simulink model "QPSK1"  (Simulink 8.0)
settings: Solver=ode45  StartTime=0.0  StopTime=12  RelTol=1e-3
libraries: commsequence2 x1, commseqgen2 x1, commutil2 x1
settings Model: Creator=Dimav  LastModifiedBy=Dimav

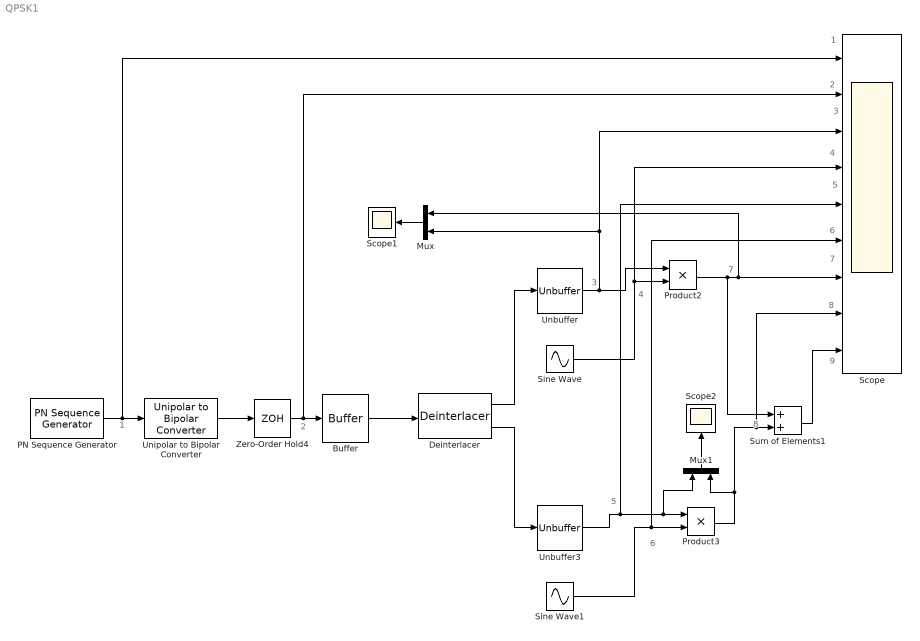
== system QPSK1 ==
  note: 8
  note: 5
  note: 5
  note: 6
  note: 6
  note: 7
  note: 7
  note: 3
  note: 4
  note: 2
  note: 1
  note: 3
  note: 8
  note: 9
  note: 1
  note: 2
  note: 4
  Buffer : Buffer  N=2  TreatMby1Signals=One channel
  Deinterlacer : commsequence2/Deinterlacer
  Mux : Mux  Inputs=2
  Mux1 : Mux  Inputs=2
  PN Sequence Generator : commseqgen2/PN Sequence Generator  poly=[1 0 0 0 0 1 1]  ini_sta=[0 0 0 0 0 1]  outBitMaskSource=Dialog parameter  shift=0  outVarSiz=off  maxOutSizeMode=Dialog parameter  maxOutSize=[10 1]  Ts=1/1200  frameBased=off  sampPerFrame=1  reset=off  bitPackedOutputs=off  outDataType=double  numPackedBits=8  bitPackDataSigned=off  bitPackedOutDType=double
  Product2 : Product  RndMeth=Zero
  Product3 : Product  RndMeth=Zero
  Scope : Scope  NumInputPorts=9
      settings: TickLabels=on  TimeRange=12  YMin=-5~-5~-5~-5~-5~-5~-5~-5~-5  YMax=5~5~5~5~5~5~5~5~5
  Scope1 : Scope
  Scope2 : Scope
      settings: SaveName=ScopeData2
  Sine Wave : Sin  Frequency=753600  Phase=-pi/2  SampleTime=0
  Sine Wave1 : Sin  Frequency=753600  SampleTime=0
  Sum of Elements1 : Sum  Inputs=2
  Unbuffer : Unbuffer  SampleBasedProcessing=Same as frame based
  Unbuffer3 : Unbuffer  SampleBasedProcessing=Same as frame based
  Unipolar to Bipolar Converter : commutil2/Unipolar to Bipolar Converter  M=2  polarity=Positive  dataType=Inherit via internal rule
  Zero-Order Hold4 : ZeroOrderHold
  wires:
  PN Sequence Generator/1 -> Scope/1, Unipolar to Bipolar Converter/1
  Unipolar to Bipolar Converter/1 -> Zero-Order Hold4/1
  Zero-Order Hold4/1 -> Scope/2, Buffer/1
  Buffer/1 -> Deinterlacer/1
  Deinterlacer/1 -> Unbuffer/1
  Deinterlacer/2 -> Unbuffer3/1
  Mux/1 -> Scope1/1
  Sine Wave1/1 -> Scope/6, Product3/2
  Unbuffer3/1 -> Scope/5, Mux1/1, Product3/1
  Mux1/1 -> Scope2/1
  Product3/1 -> Mux1/2, Scope/8, Sum of Elements1/2
  Sum of Elements1/1 -> Scope/9
  Product2/1 -> Mux/1, Scope/7, Sum of Elements1/1
  Unbuffer/1 -> Mux/2, Scope/3, Product2/1
  Sine Wave/1 -> Scope/4, Product2/2
